simulink model "AVW_b"  (Simulink 8.7)
settings: Solver=ode1  SolverMode=SingleTasking  StartTime=0.0  StopTime=500  FixedStep=0.001  RelTol=1e-3
(part 1 of 4)
settings Model: Creator=李昊泉  LastModifiedBy=user
settings DataIOCC: LimitDataPoints=off  SaveFormat=Dataset
settings DebuggingCC: UnderspecifiedInitializationDetection=Simplified  MergeDetectMultiDrivingBlocksExec=error  MultiTaskRateTransMsg=warning  SFUnexpectedBacktrackingDiag=error  SFNoUnconditionalDefaultTransitionDiag=error
settings HardwareCC: ProdBitPerPointer=64  ProdLargestAtomicFloat=Float  ProdIntDivRoundTo=Zero  ProdEndianess=LittleEndian  ProdWordSize=64  ProdHWDeviceType=Intel->x86-64 (Windows64)
settings ModelReferenceCC: PropagateSignalLabelsOutOfModel=on
settings GRTTargetCC: TargetLangStandard=C99 (ISO)  GeneratePreprocessorConditionals=Use local settings
settings ConfigComp: CovMetricSettings=dwe  CovHtmlReporting=off  CovSaveCumulativeToWorkspaceVar=off  CovSaveSingleToWorkspaceVar=off  CovModelRefEnable=off  CovExternalEMLEnable=on

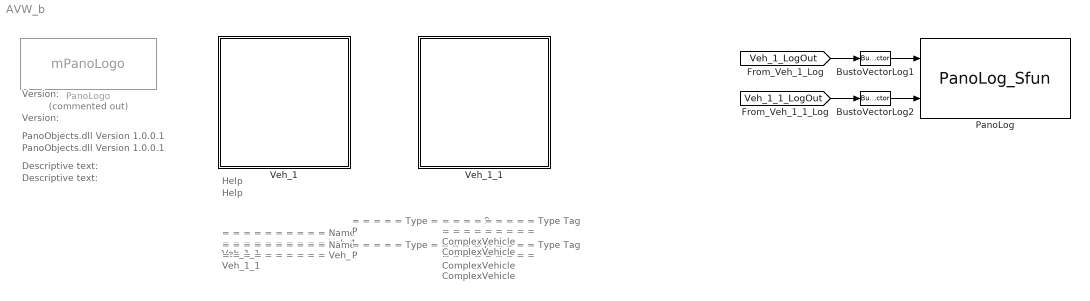
== system AVW_b ==
  note: Version:
  note: PanoObjects.dll Version 1.0.0.1
  note: Descriptive text:
  note: Help
  note: = = = = = = = = = =
      |   Name
      | = = = = = = = = = =
      |  Veh_1
      |  Veh_1_1
  note: = = = = =
      |   Type
      | = = = = =
      |   P
      |   P
  note: = = = = = = = = =
      |     Type Tag
      | = = = = = = = = =
      |  ComplexVehicle
      |  ComplexVehicle
  note: Version:
  note: PanoObjects.dll Version 1.0.0.1
  note: Descriptive text:
  note: Help
  note: = = = = = = = = = =
      |   Name
      | = = = = = = = = = =
      |  Veh_1
      |  Veh_1_1
  note: = = = = =
      |   Type
      | = = = = =
      |   P
      |   P
  note: = = = = = = = = =
      |     Type Tag
      | = = = = = = = = =
      |  ComplexVehicle
      |  ComplexVehicle
  BustoVectorLog1 : BusToVector  Tag=PanoSim_System
  BustoVectorLog2 : BusToVector  Tag=PanoSim_System
  PanoLog : S-Function  Tag=PanoSim_System  FunctionName=PanoLog_Sfun  Parameters='2','@a44ccdad-f3b7-457b-a93d-aa312d6adfaf@061ba28a-7ae2-444e-a441-87ffc9ae99f9','Matlab'  SFunctionDeploymentMode=off  EnableBusSupport=off
  PanoLogo : M-S-Function  Tag=PanoSim_System  Commented=on  FunctionName=mPanoLogo
      mask DialogControl Control2 Prompt: Welcome to use PanoSim!
      mask Display: image(imread('panosim.jpg'));
  Veh_1 : Subsystem  Tag=PanoSim_System
      mask Display: image(imread('Sedan_2.jpg'));color('white');text(0,0,'Veh_1','HorizontalAlignment','left','verticalAlignment','bottom');color('red');text(0.1,0.1,'P','HorizontalAlignment','right','verticalAlignment','top');
  Veh_1_1 : Subsystem  Tag=PanoSim_System
      mask Display: image(imread('Sedan_2.jpg'));color('white');text(0,0,'Veh_1_1','HorizontalAlignment','left','verticalAlignment','bottom');color('red');text(0.1,0.1,'P','HorizontalAlignment','right','verticalAlignment','top');
  wires:
  [Veh_1_LogOut] -> BustoVectorLog1/1
  BustoVectorLog1/1 -> PanoLog/1
  [Veh_1_1_LogOut] -> BustoVectorLog2/1
  BustoVectorLog2/1 -> PanoLog/2

== system AVW_b/Veh_1 ==
  note: = = = = = = = = = = = = = = = = = = = = = = = = = = = = = = = = =
      | English Description
      | = = = = = = = = = = = = = = = = = = = = = = = = = = = = = = = = =
      | Vehicle output bus
  note: = = = =
      | Unit
      | = = = =
  note: = = = =
      | Type
      | = = = =
      | Array
  note: = = = = = = = = = = =
      | Signal Source
      | = = = = = = = = = = =
      |  Vehicle
  note: = = = = = = = =
      | Output
      | = = = = = = = =
      |  Vehicle_out
  note: = = = = = = = = = = = = = = = = = = = = = = = = = = = = = = = = =
      | English Description
      | = = = = = = = = = = = = = = = = = = = = = = = = = = = = = = = = =
      |  throttle
      |  Gear mode, 0 neutral, 1 manual, 5 automatic ,  -1 reverse
      |  In manual mode, gear is defined by variable driver
      |  Brake master cylinder pressure
      |  Steering wheel angle
      |  wheel brake moment
      |  Wheel steering angle
  note: = = = =
      | Unit
      | = = = =
      |
      |
      |
      |  Pa
      |  rad
      |
      |  rad
  note: = = = =
      | Type
      | = = = =
      |  Single
      |  Single
      |  Single
      |  Single
      |  Single
      |  Array
      |  Array
  note: = = = = = = = = = = =
      | Signal Source
      | = = = = = = = = = = =
      |  Driver(Powertrian)
      |  Driver(Powertrian)
      |  Driver(Powertrian)
      |  Driver(Brake)
      |  Driver(Steer)
      |  Ground
      |  Ground
  note: = = = = = = = =
      | Input
      | = = = = = = = =
      |  throttle
      |  modetr
      |  geartr
      |  pcon_bk
      |  drstr_drv
      |  direc_brake
      |  direc_steer
  note: Help
  ComplexVehicleModel : Subsystem  Tag=PanoSim_System
      mask Display: image(imread('Sedan_2.jpg'));color('white');text(0,0,'Veh_1','HorizontalAlignment','left','verticalAlignment','bottom');color('red');text(0.1,0.1,'P','HorizontalAlignment','right','verticalAlignment','top');
  DriverModel : Subsystem  Tag=PanoSim_System
      mask Display: image(imread('driver.jpg'))
  Ground : Ground
  Ground1 : Ground
  Subsystem : Subsystem
  V2Sens : BusCreator  Tag=PanoSim_System  Inputs=7
  VehBusSelector1 : BusSelector  Tag=PanoSim_System  OutputSignals=Body_Out_Bus.Chassis_Motion.XO,Body_Out_Bus.Chassis_Motion.YO,Body_Out_Bus.Chassis_Motion.ZO,Body_Out_Bus.Chassis_Motion.YAW,Body_Out_Bus.Chassis_Motion.PITCH,Body_Out_Bus.Chassis_Motion.ROLL,Body_Out_Bus.Chassis_Motion.VX
  VehBusSelector2 : BusSelector  Tag=PanoSim_System  OutputSignals=Driver2Powertrain.throttle,Driver2Powertrain.modetr,Driver2Powertrain.geartr,Driver2Brake.pcon_bk,Driver2Steer.drstr_drv
  Veh_1_Sensors : Subsystem  Tag=PanoSim_System
      mask Display: image(imread('sensor.jpg'))
  tag scope: Veh_1_LogOut=global
  wires:
  Subsystem/1(PlotBuilder_out) -> [Veh_1_LogOut]
  ComplexVehicleModel/1(VehicleOut) -> Subsystem/1(VehicleDynOut), [VehicleDynOut], VehBusSelector1/1  "Vehicle_Out"
  V2Sens/1 -> [VehicleOut], Veh_1_Sensors/1(In1)
  VehBusSelector2/1 -> ComplexVehicleModel/1(Throttle)  "<throttle>"
  VehBusSelector2/5 -> ComplexVehicleModel/5(SteerAngle)  "<drstr_drv>"
  DriverModel/1(DriverOut) -> VehBusSelector2/1
  VehBusSelector1/1 -> V2Sens/1  "<XO>"
  [VehicleDynOut] -> DriverModel/1(VehicleInput)
  Ground/1 -> ComplexVehicleModel/6(Direct Brake)
  VehBusSelector1/3 -> V2Sens/3  "<ZO>"
  VehBusSelector1/4 -> V2Sens/4  "<YAW>"
  VehBusSelector1/2 -> V2Sens/2  "<YO>"
  VehBusSelector1/7 -> V2Sens/7  "<VX>"
  Ground1/1 -> ComplexVehicleModel/7(Direct Steer)
  VehBusSelector1/6 -> V2Sens/6  "<ROLL>"
  VehBusSelector2/4 -> ComplexVehicleModel/4(BrakeControl)  "<pcon_bk>"
  VehBusSelector1/5 -> V2Sens/5  "<PITCH>"
  VehBusSelector2/3 -> ComplexVehicleModel/3(Gear)  "<geartr>"
  VehBusSelector2/2 -> ComplexVehicleModel/2(TransMode)  "<modetr>"

== system AVW_b/Veh_1_1 ==
  note: = = = = = = = = = = = = = = = = = = = = = = = = = = = = = = = = =
      | English Description
      | = = = = = = = = = = = = = = = = = = = = = = = = = = = = = = = = =
      | Vehicle output bus
  note: = = = =
      | Unit
      | = = = =
  note: = = = =
      | Type
      | = = = =
      | Array
  note: = = = = = = = = = = =
      | Signal Source
      | = = = = = = = = = = =
      |  Vehicle
  note: = = = = = = = =
      | Output
      | = = = = = = = =
      |  Vehicle_out
  note: = = = = = = = = = = = = = = = = = = = = = = = = = = = = = = = = =
      | English Description
      | = = = = = = = = = = = = = = = = = = = = = = = = = = = = = = = = =
      |  throttle
      |  Gear mode, 0 neutral, 1 manual, 5 automatic ,  -1 reverse
      |  In manual mode, gear is defined by variable driver
      |  Brake master cylinder pressure
      |  Steering wheel angle
      |  wheel brake moment
      |  Wheel steering angle
  note: = = = =
      | Unit
      | = = = =
      |
      |
      |
      |  Pa
      |  rad
      |
      |  rad
  note: = = = =
      | Type
      | = = = =
      |  Single
      |  Single
      |  Single
      |  Single
      |  Single
      |  Array
      |  Array
  note: = = = = = = = = = = =
      | Signal Source
      | = = = = = = = = = = =
      |  Driver(Powertrian)
      |  Driver(Powertrian)
      |  Driver(Powertrian)
      |  Driver(Brake)
      |  Driver(Steer)
      |  Ground
      |  Ground
  note: = = = = = = = =
      | Input
      | = = = = = = = =
      |  throttle
      |  modetr
      |  geartr
      |  pcon_bk
      |  drstr_drv
      |  direc_brake
      |  direc_steer
  note: Help
  ComplexVehicleModel : Subsystem  Tag=PanoSim_System
      mask Display: image(imread('Sedan_2.jpg'));color('white');text(0,0,'Veh_1_1','HorizontalAlignment','left','verticalAlignment','bottom');color('red');text(0.1,0.1,'P','HorizontalAlignment','right','verticalAlignment','top');
  DriverModel : Subsystem  Tag=PanoSim_System
      mask Display: image(imread('driver.jpg'))
  Ground : Ground
  Ground1 : Ground
  Subsystem : Subsystem
  V2Sens : BusCreator  Tag=PanoSim_System  Inputs=7
  VehBusSelector1 : BusSelector  Tag=PanoSim_System  OutputSignals=Body_Out_Bus.Chassis_Motion.XO,Body_Out_Bus.Chassis_Motion.YO,Body_Out_Bus.Chassis_Motion.ZO,Body_Out_Bus.Chassis_Motion.YAW,Body_Out_Bus.Chassis_Motion.PITCH,Body_Out_Bus.Chassis_Motion.ROLL,Body_Out_Bus.Chassis_Motion.VX
  VehBusSelector2 : BusSelector  Tag=PanoSim_System  OutputSignals=Driver2Powertrain.throttle,Driver2Powertrain.modetr,Driver2Powertrain.geartr,Driver2Brake.pcon_bk,Driver2Steer.drstr_drv
  Veh_1_1_Sensors : Subsystem  Tag=PanoSim_System
      mask Display: image(imread('sensor.jpg'))
  tag scope: Veh_1_1_LogOut=global
  wires:
  Subsystem/1(PlotBuilder_out) -> [Veh_1_1_LogOut]
  ComplexVehicleModel/1(VehicleOut) -> Subsystem/1(VehicleDynOut), [VehicleDynOut], VehBusSelector1/1  "Vehicle_Out"
  V2Sens/1 -> [VehicleOut], Veh_1_1_Sensors/1(In1)
  VehBusSelector2/1 -> ComplexVehicleModel/1(Throttle)  "<throttle>"
  VehBusSelector2/5 -> ComplexVehicleModel/5(SteerAngle)  "<drstr_drv>"
  DriverModel/1(DriverOut) -> VehBusSelector2/1
  VehBusSelector1/1 -> V2Sens/1  "<XO>"
  [VehicleDynOut] -> DriverModel/1(VehicleInput)
  Ground/1 -> ComplexVehicleModel/6(Direct Brake)
  VehBusSelector1/3 -> V2Sens/3  "<ZO>"
  VehBusSelector1/4 -> V2Sens/4  "<YAW>"
  VehBusSelector1/2 -> V2Sens/2  "<YO>"
  VehBusSelector1/7 -> V2Sens/7  "<VX>"
  Ground1/1 -> ComplexVehicleModel/7(Direct Steer)
  VehBusSelector1/6 -> V2Sens/6  "<ROLL>"
  VehBusSelector2/4 -> ComplexVehicleModel/4(BrakeControl)  "<pcon_bk>"
  VehBusSelector1/5 -> V2Sens/5  "<PITCH>"
  VehBusSelector2/3 -> ComplexVehicleModel/3(Gear)  "<geartr>"
  VehBusSelector2/2 -> ComplexVehicleModel/2(TransMode)  "<modetr>"

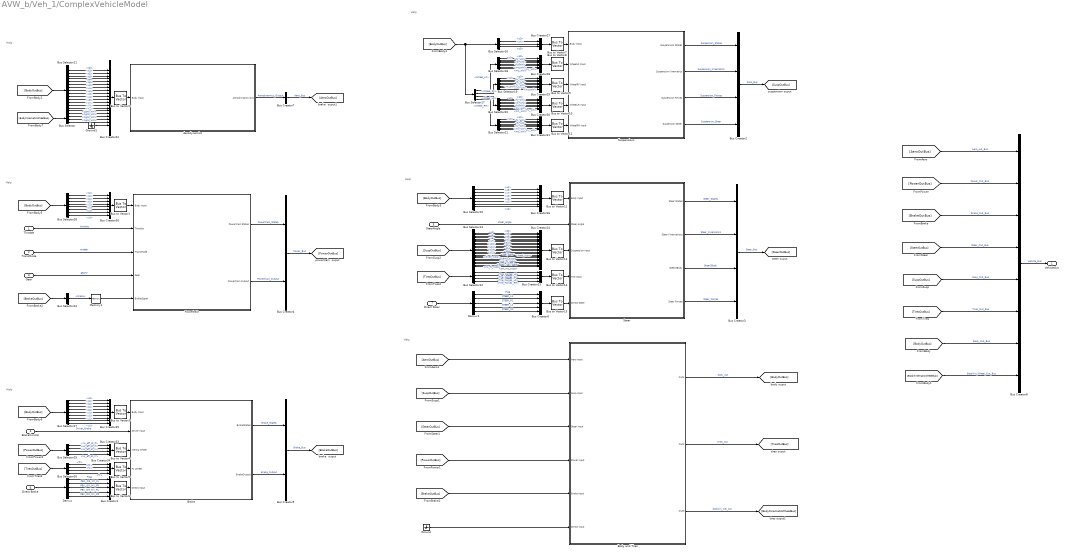
== system AVW_b/Veh_1/ComplexVehicleModel ==
  note: Help
  note: Help
  note: Help
  note: Help
  note: Help
  note: Help
  Throttle : Inport
  TransMode : Inport  Port=2
  Gear : Inport  Port=3
  BrakeControl : Inport  Port=4
  SteerAngle : Inport  Port=5
  Direct Brake : Inport  Port=6
  Direct Steer : Inport  Port=7
  Aerodynamics : Subsystem
  Body and Tires : Subsystem
  Brake : Subsystem
  Bus Creator1 : BusCreator  Inputs=5
  Bus Creator{2..3,23,33..34} (5 alike) : BusCreator  Inputs=4
  Bus Creator22 : BusCreator  Inputs=20
  Bus Creator24 : BusCreator  Inputs=24
  Bus Creator26 : BusCreator  Inputs=7
  Bus Creator27 : BusCreator  Inputs=3
  Bus Creator{8,28..31,36} (6 alike) : BusCreator  Inputs=8
  Bus Creator35 : BusCreator  Inputs=9
  Bus Creator4 : BusCreator  Inputs=2
  Bus Creator5 : BusCreator  Inputs=2
  Bus Creator6 : BusCreator  Inputs=5
  Bus Creator7 : BusCreator  Inputs=1
  Bus Selector : BusSelector  OutputSignals=bodykin_whl_out_lf.zgnd_whl,bodykin_whl_out_rf.zgnd_whl,bodykin_whl_out_lr.zgnd_whl,bodykin_whl_out_rr.zgnd_whl
  Bus Selector11 : BusSelector  OutputSignals=Chassi_States.q0,Chassi_States.q1,Chassi_States.q2,Chassi_States.q3,Chassi_States.q4,Chassi_States.q5,Chassi_States.u0,Chassi_States.u1,Chassi_States.u2,Chassi_States.u3,Chassi_States.u4,Chassi_States.u5,Chassis_Motion.VX,Chassis_Motion.VY,Chassis_Motion.VZ
  Bus Selector12 : BusSelector  OutputSignals=Tire_Forces_LF,Tire_Forces_RF,Tire_Forces_LR,Tire_Forces_RR
  Bus Selector13 : BusSelector  OutputSignals=Suspension_States.q2,Suspension_States.u2,Suspension_States.q3,Suspension_States.u3,Suspension_States.q6,Suspension_States.u6,Suspension_States.q7,Suspension_States.u7,Suspension_States.q10,Suspension_States.u10,Suspension_States.q11,Suspension_States.u11,Suspension_States.q14,Suspension_States.u14,Suspension_States.q15,Suspension_States.u15,Suspension_Kinematics.toe_susp,Suspension_Kinematics.toed_susp,Suspension_Kinematics.dived_susp,Suspension_Kinematics.camd_susp,Suspension_Kinematics.dcam_con_susp,Suspension_Steer.sw_fx_susp,Suspension_Steer.sw_fy_susp,Suspension_Steer.sw_mz_susp
  Bus Selector15 : BusSelector  OutputSignals=Chassi_States.u0,Chassi_States.u6,Chassi_States.u7,Wheel_LF.u0,Wheel_RF.u0,Wheel_LR.u0,Wheel_RR.u0
  Bus Selector16 : BusSelector  OutputSignals=Chassi_States.u3,Chassi_States.u4,Chassi_States.u5
  Bus Selector17 : BusSelector  OutputSignals=Wheel_LF,Wheel_RF,Wheel_LR,Wheel_RR
  Bus Selector{18..21} (4 alike) : BusSelector  OutputSignals=q0,u0,fx_whl,fy_whl,fz_whl,mx_whl,my_whl,mz_whl
  Bus Selector23 : BusSelector  OutputSignals=Brake_Output.brake
  Bus Selector25 : BusSelector  OutputSignals=Powertrain_Output.iw_eff_pt_lf,Powertrain_Output.iw_eff_pt_rf,Powertrain_Output.iw_eff_pt_lr,Powertrain_Output.iw_eff_pt_rr
  Bus Selector26 : BusSelector  OutputSignals=Tire_Forces_LF.fz,Tire_Forces_RF.fz,Tire_Forces_LR.fz,Tire_Forces_RR.fz
  Bus Selector27 : BusSelector  OutputSignals=Chassi_States.u0,Wheel_LF.q1,Wheel_RF.q1,Wheel_LR.q1,Wheel_RR.q1,Wheel_LF.u1,Wheel_RF.u1,Wheel_LR.u1,Wheel_RR.u1
  Bus Selector28 : BusSelector  OutputSignals=Wheel_LF.q1,Wheel_RF.q1,Wheel_LR.q1,Wheel_RR.q1,Wheel_LF.u1,Wheel_RF.u1,Wheel_LR.u1,Wheel_RR.u1
  Bus to Vector{1..15} (15 alike) : BusToVector
  Demux : Demux  Outputs=5
  Demux1 : Demux  Outputs=5
  Ground : Ground
  Ground1 : Ground
  Memory1 : Memory
  Powertrain : Subsystem
  Steer : Subsystem
  Suspensions : Subsystem
  VehicleOut : Outport
  wires:
  Ground/1 -> Body and Tires/6(Direct Input)
  Bus Selector13/24 -> Bus Creator24/24  "<sw_mz_susp>"
  Bus Selector13/23 -> Bus Creator24/23  "<sw_fy_susp>"
  Bus Selector13/22 -> Bus Creator24/22  "<sw_fx_susp>"
  Bus Selector13/21 -> Bus Creator24/21  "<dcam_con_susp>"
  Bus Selector13/20 -> Bus Creator24/20  "<camd_susp>"
  Bus Selector13/19 -> Bus Creator24/19  "<dived_susp>"
  Bus Selector13/18 -> Bus Creator24/18  "<toed_susp>"
  Bus Selector13/17 -> Bus Creator24/17  "<toe_susp>"
  Bus Selector13/16 -> Bus Creator24/16  "<u15>"
  Bus Selector13/15 -> Bus Creator24/15  "<q15>"
  Bus Selector13/14 -> Bus Creator24/14  "<u14>"
  Bus Selector13/13 -> Bus Creator24/13  "<q14>"
  Bus Selector13/12 -> Bus Creator24/12  "<u11>"
  Bus Selector13/11 -> Bus Creator24/11  "<q11>"
  Bus Selector13/10 -> Bus Creator24/10  "<u10>"
  Bus Selector13/9 -> Bus Creator24/9  "<q10>"
  Bus Selector13/8 -> Bus Creator24/8  "<u7>"
  Bus Selector13/7 -> Bus Creator24/7  "<q7>"
  Bus Selector13/6 -> Bus Creator24/6  "<u6>"
  Bus Selector13/5 -> Bus Creator24/5  "<q6>"
  Bus Selector13/4 -> Bus Creator24/4  "<u3>"
  Bus Selector13/3 -> Bus Creator24/3  "<q3>"
  Bus Selector13/2 -> Bus Creator24/2  "<u2>"
  Bus Selector13/1 -> Bus Creator24/1  "<q2>"
  Demux1/5 -> Bus Creator6/5  "STEER_R2"
  Demux1/4 -> Bus Creator6/4  "STEER_L2"
  Demux1/3 -> Bus Creator6/3  "STEER_R1"
  Demux1/2 -> Bus Creator6/2  "STEER_L1"
  Demux1/1 -> Bus Creator6/1  "Flag"
  Direct Steer/1 -> Demux1/1
  Bus Creator6/1 -> Bus to Vector15/1
  Demux/5 -> Bus Creator1/5  "PBK_OR_MY_RR"
  Demux/4 -> Bus Creator1/4  "PBK_OR_MY_RL"
  Demux/3 -> Bus Creator1/3  "PBK_OR_MY_FR"
  Demux/2 -> Bus Creator1/2  "PBK_OR_MY_FL"
  Demux/1 -> Bus Creator1/1  "Flag"
  Direct Brake/1 -> Demux/1
  SteerAngle/1 -> Steer/2(Steer Angle)  "steer_angle"
  [TiresOutBus] -> Bus Creator8/6  "Tires_Out_Bus"
  [SuspOutBus] -> Bus Creator8/5  "Susp_Out_Bus"
  [SteerOutBus] -> Bus Creator8/4  "Steer_Out_Bus"
  [BrakeOutBus] -> Bus Creator8/3  "Brake_Out_Bus"
  [PowerOutBus] -> Bus Creator8/2  "Power_Out_BUs"
  [AeroOutBus] -> Bus Creator8/1  "Aero_out_Bus"
  Suspensions/4(Suspension Steer) -> Bus Creator2/4  "Suspension_Steer"
  Suspensions/3(Suspension Forces) -> Bus Creator2/3  "Suspension_Forces"
  Suspensions/1(Suspensions States) -> Bus Creator2/1  "Suspension_States"
  Suspensions/2(Suspension Kinematics) -> Bus Creator2/2  "Suspension_Kinematics"
  Bus Creator2/1 -> [SuspOutBus]  "Susp_Bus"
  Steer/1(Steer States) -> Bus Creator3/1  "Steer_States"
  Steer/2(Steer Kinematiocs) -> Bus Creator3/2  "Steer_Kinematics"
  Steer/3(Steer2Body) -> Bus Creator3/3  "Steer2Body"
  Steer/4(Steer Forces) -> Bus Creator3/4  "Steer_Forces"
  Bus Creator3/1 -> [SteerOutBus]  "Steer_Bus"
  Powertrain/1(Powertrain States) -> Bus Creator4/1  "Powertrain_States"
  Powertrain/2(Powertrain Output) -> Bus Creator4/2  "Powertrain_Output"
  Bus Creator4/1 -> [PowerOutBus]  "Power_Bus"
  Brake/1(BrakeStates) -> Bus Creator5/1  "Brake_States"
  Brake/2(BrakeOutput) -> Bus Creator5/2  "Brake_Output"
  Bus Creator5/1 -> [BrakeOutBus]  "Brake_Bus"
  Aerodynamics/1(Aerodymatics Out) -> Bus Creator7/1  "Aerodynamics_Output"
  Bus Creator7/1 -> [AeroOutBus]  "Aero_Bus"
  Bus Creator8/1 -> VehicleOut/1  "Vehicle_Bus"
  [BodyOutBus] -> Bus Creator8/7  "Body_Out_Bus"
  [BodyOutBus] -> Bus Selector11/1
  [TiresOutBus] -> Bus Selector12/1
  Bus Selector12/1 -> Bus Creator23/1  "<Tire_Forces_LF>"
  Bus Selector12/2 -> Bus Creator23/2  "<Tire_Forces_RF>"
  Bus Selector12/3 -> Bus Creator23/3  "<Tire_Forces_LR>"
  Bus Selector12/4 -> Bus Creator23/4  "<Tire_Forces_RR>"
  [SuspOutBus] -> Bus Selector13/1
  Bus Creator24/1 -> Bus to Vector13/1
  [BodyOutBus] -> Bus Selector15/1
  Bus Selector15/1 -> Bus Creator26/1  "<u0>"
  Bus Selector15/2 -> Bus Creator26/2  "<u6>"
  Bus Selector15/3 -> Bus Creator26/3  "<u7>"
  Bus Selector15/4 -> Bus Creator26/4  "<u0>"
  Bus Selector15/5 -> Bus Creator26/5  "<u0>"
  Bus Selector15/6 -> Bus Creator26/6  "<u0>"
  Bus Selector15/7 -> Bus Creator26/7  "<u0>"
  Bus Selector16/1 -> Bus Creator27/1  "<u3>"
  Bus Selector16/2 -> Bus Creator27/2  "<u4>"
  Bus Selector16/3 -> Bus Creator27/3  "<u5>"
  Bus Creator27/1 -> Bus to Vector7/1
  Bus Selector17/1 -> Bus Selector18/1  "<Wheel_LF>"
  Bus Selector18/1 -> Bus Creator28/1  "<q0>"
  Bus Selector18/2 -> Bus Creator28/2  "<u0>"
  Bus Selector18/3 -> Bus Creator28/3  "<fx_whl>"
  Bus Selector18/4 -> Bus Creator28/4  "<fy_whl>"
  Bus Selector18/5 -> Bus Creator28/5  "<fz_whl>"
  Bus Selector18/6 -> Bus Creator28/6  "<mx_whl>"
  Bus Selector18/7 -> Bus Creator28/7  "<my_whl>"
  Bus Selector18/8 -> Bus Creator28/8  "<mz_whl>"
  Bus Selector19/1 -> Bus Creator29/1  "<q0>"
  Bus Selector19/2 -> Bus Creator29/2  "<u0>"
  Bus Selector19/3 -> Bus Creator29/3  "<fx_whl>"
  Bus Selector19/4 -> Bus Creator29/4  "<fy_whl>"
  Bus Selector19/5 -> Bus Creator29/5  "<fz_whl>"
  Bus Selector19/6 -> Bus Creator29/6  "<mx_whl>"
  Bus Selector19/7 -> Bus Creator29/7  "<my_whl>"
  Bus Selector19/8 -> Bus Creator29/8  "<mz_whl>"
  Bus Selector20/1 -> Bus Creator30/1  "<q0>"
  Bus Selector20/2 -> Bus Creator30/2  "<u0>"
  Bus Selector20/3 -> Bus Creator30/3  "<fx_whl>"
  Bus Selector20/4 -> Bus Creator30/4  "<fy_whl>"
  Bus Selector20/5 -> Bus Creator30/5  "<fz_whl>"
  Bus Selector20/6 -> Bus Creator30/6  "<mx_whl>"
  Bus Selector20/7 -> Bus Creator30/7  "<my_whl>"
  Bus Selector20/8 -> Bus Creator30/8  "<mz_whl>"
  Bus Selector21/1 -> Bus Creator31/1  "<q0>"
  Bus Selector21/2 -> Bus Creator31/2  "<u0>"
  Bus Selector21/3 -> Bus Creator31/3  "<fx_whl>"
  Bus Selector21/4 -> Bus Creator31/4  "<fy_whl>"
  Bus Selector21/5 -> Bus Creator31/5  "<fz_whl>"
  Bus Selector21/6 -> Bus Creator31/6  "<mx_whl>"
  Bus Selector21/7 -> Bus Creator31/7  "<my_whl>"
  Bus Selector21/8 -> Bus Creator31/8  "<mz_whl>"
  Bus Selector17/2 -> Bus Selector19/1  "<Wheel_RF>"
  Bus Selector17/3 -> Bus Selector20/1  "<Wheel_LR>"
  Bus Selector17/4 -> Bus Selector21/1  "<Wheel_RR>"
  Bus Creator28/1 -> Bus to Vector8/1
  Bus Creator29/1 -> Bus to Vector9/1
  Bus Creator30/1 -> Bus to Vector10/1
  Bus Creator31/1 -> Bus to Vector11/1
  Throttle/1 -> Powertrain/2(Throttle)  "throttle"
  TransMode/1 -> Powertrain/3(TransMode)  "modetr"
  Gear/1 -> Powertrain/4(Gear)  "geartr"
  [BrakeOutBus] -> Bus Selector23/1
  BrakeControl/1 -> Brake/2(Driver Input)  "Driver_Brake"
  [PowerOutBus] -> Bus Selector25/1
  Bus Selector25/1 -> Bus Creator33/1  "<iw_eff_pt_lf>"
  Bus Selector25/2 -> Bus Creator33/2  "<iw_eff_pt_rf>"
  Bus Selector25/3 -> Bus Creator33/3  "<iw_eff_pt_lr>"
  Bus Selector25/4 -> Bus Creator33/4  "<iw_eff_pt_rr>"
  [TiresOutBus] -> Bus Selector26/1
  Bus Selector26/1 -> Bus Creator34/1  "<fz>"
  Bus Selector26/2 -> Bus Creator34/2  "<fz>"
  Bus Selector26/3 -> Bus Creator34/3  "<fz>"
  Bus Selector26/4 -> Bus Creator34/4  "<fz>"
  [BodyOutBus] -> Bus Selector27/1
  Bus Selector27/1 -> Bus Creator35/1  "<u0>"
  Bus Selector27/2 -> Bus Creator35/2  "<q1>"
  Bus Selector27/3 -> Bus Creator35/3  "<q1>"
  Bus Selector27/4 -> Bus Creator35/4  "<q1>"
  Bus Selector27/5 -> Bus Creator35/5  "<q1>"
  Bus Selector27/6 -> Bus Creator35/6  "<u1>"
  Bus Selector27/7 -> Bus Creator35/7  "<u1>"
  Bus Selector27/8 -> Bus Creator35/8  "<u1>"
  Bus Selector27/9 -> Bus Creator35/9  "<u1>"
  [BodyOutBus] -> Bus Selector28/1
  Bus Selector28/1 -> Bus Creator36/1  "<q1>"
  Bus Selector28/2 -> Bus Creator36/2  "<q1>"
  Bus Selector28/3 -> Bus Creator36/3  "<q1>"
  Bus Selector28/4 -> Bus Creator36/4  "<q1>"
  Bus Selector28/5 -> Bus Creator36/5  "<u1>"
  Bus Selector28/6 -> Bus Creator36/6  "<u1>"
  Bus Selector28/7 -> Bus Creator36/7  "<u1>"
  Bus Selector28/8 -> Bus Creator36/8  "<u1>"
  Bus Selector11/1 -> Bus Creator22/1  "<q0>"
  Bus Selector11/2 -> Bus Creator22/2  "<q1>"
  Bus Selector11/3 -> Bus Creator22/3  "<q2>"
  Bus Selector11/4 -> Bus Creator22/4  "<q3>"
  Bus Selector11/5 -> Bus Creator22/5  "<q4>"
  Bus Selector11/6 -> Bus Creator22/6  "<q5>"
  Bus Selector11/7 -> Bus Creator22/7  "<u0>"
  Bus Selector11/8 -> Bus Creator22/8  "<u1>"
  Bus Selector11/9 -> Bus Creator22/9  "<u2>"
  Bus Selector11/10 -> Bus Creator22/10  "<u3>"
  Bus Selector11/11 -> Bus Creator22/11  "<u4>"
  Bus Selector11/12 -> Bus Creator22/12  "<u5>"
  Bus Selector11/13 -> Bus Creator22/13  "<VX>"
  Bus Selector11/14 -> Bus Creator22/14  "<VY>"
  Bus Selector11/15 -> Bus Creator22/15  "<VZ>"
  Ground1/1 -> Bus Creator22/20
  [SteerOutBus] -> Body and Tires/3(Steer Input)
  [PowerOutBus] -> Body and Tires/4(Power Input)
  Body and Tires/1(Out1) -> [BodyOutBus]  "body_out"
  Body and Tires/2(Out2) -> [TiresOutBus]  "tires_out"
  [AeroOutBus] -> Body and Tires/1(Aero Input)
  [SuspOutBus] -> Body and Tires/2(Susp Input)
  Bus Selector23/1 -> Memory1/1  "<brake>"
  Memory1/1 -> Powertrain/5(BrakeSignal)
  Bus Creator26/1 -> Bus to Vector12/1
  Bus Creator23/1 -> Bus to Vector14/1
  Bus Creator36/1 -> Bus to Vector1/1
  [BodyOutBus] -> Bus Selector16/1, Bus Selector17/1
  [BrakeOutBus] -> Body and Tires/5(Brake Input)
  Body and Tires/3(Out3) -> [BodyKinematicWheelBus]  "bodykin_wel_out"
  [BodyKinematicWheelBus] -> Bus Creator8/8  "BodyKin_Wheel_Out_Bus"
  [BodyKinematicWheelBus] -> Bus Selector/1
  Bus Selector/1 -> Bus Creator22/16  "<zgnd_whl>"
  Bus Selector/2 -> Bus Creator22/17  "<zgnd_whl>"
  Bus Selector/3 -> Bus Creator22/18  "<zgnd_whl>"
  Bus Selector/4 -> Bus Creator22/19  "<zgnd_whl>"
  Bus Creator22/1 -> Bus to Vector2/1
  Bus to Vector2/1 -> Aerodynamics/1(Body Input)
  Bus to Vector1/1 -> Powertrain/1(Body Input)
  Bus Creator35/1 -> Bus to Vector3/1
  Bus to Vector3/1 -> Brake/1(Body Input)
  Bus Creator33/1 -> Bus to Vector4/1
  Bus to Vector4/1 -> Brake/3(Inertia Wheel)
  Bus Creator34/1 -> Bus to Vector5/1
  Bus to Vector5/1 -> Brake/4(Fz Wheel)
  Bus Creator1/1 -> Bus to Vector6/1
  Bus to Vector6/1 -> Brake/5(Direct Input)
  Bus to Vector7/1 -> Suspensions/1(Body Input)
  Bus to Vector8/1 -> Suspensions/2(WheelLF Input)
  Bus to Vector9/1 -> Suspensions/3(WheelRF Input)
  Bus to Vector10/1 -> Suspensions/4(WheelLR Input)
  Bus to Vector11/1 -> Suspensions/5(WheelRR Input)
  Bus to Vector12/1 -> Steer/1(Body Input)
  Bus to Vector13/1 -> Steer/3(Suspension Input)
  Bus to Vector14/1 -> Steer/4(Tire Input)
  Bus to Vector15/1 -> Steer/5(Direct Steer)

== system AVW_b/Veh_1/DriverModel ==
  note: Help
  VehicleInput : Inport
  Bus Creator37 : BusCreator  Inputs=10
  Bus Creator38 : BusCreator  Inputs=2
  Bus Creator39 : BusCreator  Inputs=2
  Bus Creator6 : BusCreator  Inputs=4
  Bus Selector : BusSelector  OutputSignals=Body_Out_Bus,Steer_Out_Bus,Power_Out_BUs,Brake_Out_Bus
  Bus Selector29 : BusSelector  OutputSignals=Chassi_States.q0,Chassi_States.q1,Chassi_States.q3,Chassi_States.u0,Chassi_States.u1,Chassi_States.u3,Wheel_LF.u1,Wheel_RF.u1,Wheel_LR.u1,Wheel_RR.u1
  Bus Selector30 : BusSelector  OutputSignals=Steer_Kinematics.str_sus_f,Steer_Kinematics.str_sus_r
  Bus Selector31 : BusSelector  OutputSignals=Powertrain_Output.av_eng,Powertrain_Output.aa_eng
  Bus Selector32 : BusSelector  OutputSignals=Brake_Output.turn_off
  Driver : Subsystem
  DriverOut : Outport
  wires:
  Bus Creator6/1 -> DriverOut/1  "Driver_Bus"
  Bus Creator39/1 -> Driver/3(Engine Input)
  Bus Selector31/2 -> Bus Creator39/2  "<aa_eng>"
  Bus Selector31/1 -> Bus Creator39/1  "<av_eng>"
  Bus Selector/3 -> Bus Selector31/1  "<Power_Out_BUs>"
  Bus Selector32/1 -> Driver/4(Brake Input)  "<turn_off>"
  Bus Creator38/1 -> Driver/2(Steer Input)
  Bus Selector30/2 -> Bus Creator38/2  "<str_sus_r>"
  Bus Selector30/1 -> Bus Creator38/1  "<str_sus_f>"
  Bus Selector/2 -> Bus Selector30/1  "<Steer_Out_Bus>"
  Bus Selector29/10 -> Bus Creator37/10  "<u1>"
  Bus Selector29/9 -> Bus Creator37/9  "<u1>"
  Bus Selector29/8 -> Bus Creator37/8  "<u1>"
  Bus Selector29/7 -> Bus Creator37/7  "<u1>"
  Bus Selector29/6 -> Bus Creator37/6  "<u3>"
  Bus Selector29/5 -> Bus Creator37/5  "<u1>"
  Bus Selector29/4 -> Bus Creator37/4  "<u0>"
  Bus Selector29/3 -> Bus Creator37/3  "<q3>"
  Bus Selector29/2 -> Bus Creator37/2  "<q1>"
  Bus Selector29/1 -> Bus Creator37/1  "<q0>"
  Bus Creator37/1 -> Driver/1(Body Input)
  Bus Selector/1 -> Bus Selector29/1  "<Body_Out_Bus>"
  Driver/4(Driver_Brake) -> Bus Creator6/4
  Driver/3(Driver_Powertrain) -> Bus Creator6/3
  Driver/2(Driver_Steer) -> Bus Creator6/2
  Driver/1(Driver_States) -> Bus Creator6/1
  VehicleInput/1 -> Bus Selector/1
  Bus Selector/4 -> Bus Selector32/1  "<Brake_Out_Bus>"

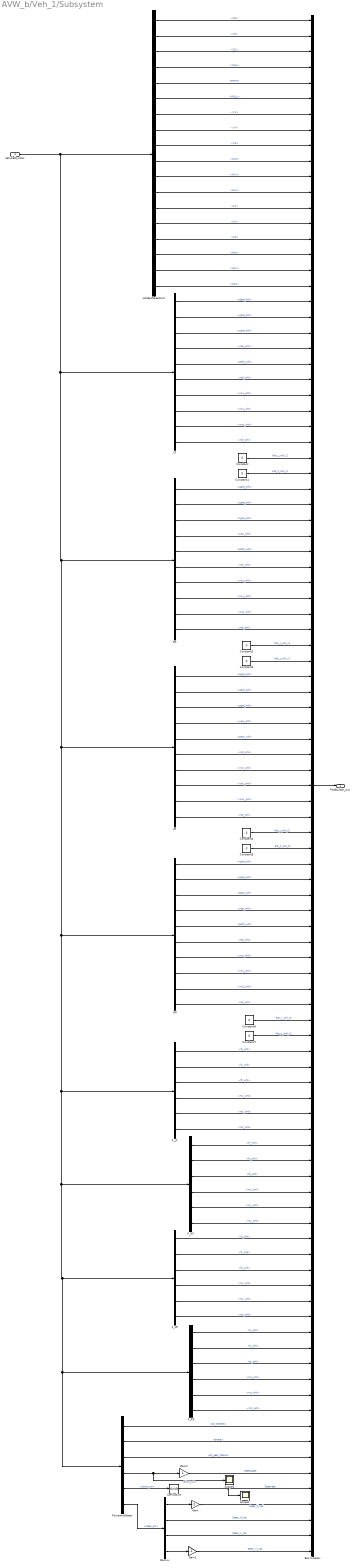
== system AVW_b/Veh_1/Subsystem ==
  VehicleDynOut : Inport
  Bus Creator : BusCreator  Inputs=99
  Constant{,1..7} (8 alike) : Constant  Value=0
  Demux : Demux
  Derivative : Derivative
  F_LF : BusSelector  Tag=PanoSim_System  OutputSignals=Body_Out_Bus.Wheel_LF.fx_whl,Body_Out_Bus.Wheel_LF.fy_whl,Body_Out_Bus.Wheel_LF.fz_whl,Body_Out_Bus.Wheel_LF.mx_whl,Body_Out_Bus.Wheel_LF.my_whl,Body_Out_Bus.Wheel_LF.mz_whl
  F_LR : BusSelector  Tag=PanoSim_System  OutputSignals=Body_Out_Bus.Wheel_LR.fx_whl,Body_Out_Bus.Wheel_LR.fy_whl,Body_Out_Bus.Wheel_LR.fz_whl,Body_Out_Bus.Wheel_LR.mx_whl,Body_Out_Bus.Wheel_LR.my_whl,Body_Out_Bus.Wheel_LR.mz_whl
  F_RF : BusSelector  Tag=PanoSim_System  OutputSignals=Body_Out_Bus.Wheel_RF.fx_whl,Body_Out_Bus.Wheel_RF.fy_whl,Body_Out_Bus.Wheel_RF.fz_whl,Body_Out_Bus.Wheel_RF.mx_whl,Body_Out_Bus.Wheel_RF.my_whl,Body_Out_Bus.Wheel_RF.mz_whl
  F_RR : BusSelector  Tag=PanoSim_System  OutputSignals=Body_Out_Bus.Wheel_RR.fx_whl,Body_Out_Bus.Wheel_RR.fy_whl,Body_Out_Bus.Wheel_RR.fz_whl,Body_Out_Bus.Wheel_RR.mx_whl,Body_Out_Bus.Wheel_RR.my_whl,Body_Out_Bus.Wheel_RR.mz_whl
  Gain : Gain  Gain=-1
  Gain1 : Gain  Gain=-1
  Gain2 : Gain
  LF : BusSelector  Tag=PanoSim_System  OutputSignals=BodyKin_Wheel_Out_Bus.bodykin_whl_out_lf.xgnd_whl,BodyKin_Wheel_Out_Bus.bodykin_whl_out_lf.ygnd_whl,BodyKin_Wheel_Out_Bus.bodykin_whl_out_lf.zgnd_whl,BodyKin_Wheel_Out_Bus.bodykin_whl_out_lf.yaw_whl,BodyKin_Wheel_Out_Bus.bodykin_whl_out_lf.pitch_whl,BodyKin_Wheel_Out_Bus.bodykin_whl_out_lf.roll_whl,BodyKin_Wheel_Out_Bus.bodykin_whl_out_lf.vwx_whl,BodyKin_Wheel_Out_Bus.bodykin_whl_out_lf.vwy_whl,BodyKin_Wheel_Out_Bus.bodykin_whl_out_lf.vwz_whl,BodyKin_Wheel_Out_Bus.bodykin_whl_out_lf.rot_whl
  LR : BusSelector  Tag=PanoSim_System  OutputSignals=BodyKin_Wheel_Out_Bus.bodykin_whl_out_lr.xgnd_whl,BodyKin_Wheel_Out_Bus.bodykin_whl_out_lr.ygnd_whl,BodyKin_Wheel_Out_Bus.bodykin_whl_out_lr.zgnd_whl,BodyKin_Wheel_Out_Bus.bodykin_whl_out_lr.yaw_whl,BodyKin_Wheel_Out_Bus.bodykin_whl_out_lr.pitch_whl,BodyKin_Wheel_Out_Bus.bodykin_whl_out_lr.roll_whl,BodyKin_Wheel_Out_Bus.bodykin_whl_out_lr.vwx_whl,BodyKin_Wheel_Out_Bus.bodykin_whl_out_lr.vwy_whl,BodyKin_Wheel_Out_Bus.bodykin_whl_out_lr.vwz_whl,BodyKin_Wheel_Out_Bus.bodykin_whl_out_lr.rot_whl
  PowerandSteer : BusSelector  Tag=PanoSim_System  OutputSignals=Power_Out_BUs.Powertrain_Output.pt_throttle,Brake_Out_Bus.Brake_Output.brake,Power_Out_BUs.Powertrain_Output.pt_gear_status,Steer_Out_Bus.Steer_Kinematics.strav_sw,Steer_Out_Bus.Steer_Kinematics.strav_sw,Steer_Out_Bus.Steer_Kinematics.steer_str
  RF : BusSelector  Tag=PanoSim_System  OutputSignals=BodyKin_Wheel_Out_Bus.bodykin_whl_out_rf.xgnd_whl,BodyKin_Wheel_Out_Bus.bodykin_whl_out_rf.ygnd_whl,BodyKin_Wheel_Out_Bus.bodykin_whl_out_rf.zgnd_whl,BodyKin_Wheel_Out_Bus.bodykin_whl_out_rf.yaw_whl,BodyKin_Wheel_Out_Bus.bodykin_whl_out_rf.pitch_whl,BodyKin_Wheel_Out_Bus.bodykin_whl_out_rf.roll_whl,BodyKin_Wheel_Out_Bus.bodykin_whl_out_rf.vwx_whl,BodyKin_Wheel_Out_Bus.bodykin_whl_out_rf.vwy_whl,BodyKin_Wheel_Out_Bus.bodykin_whl_out_rf.vwz_whl,BodyKin_Wheel_Out_Bus.bodykin_whl_out_rf.rot_whl
  RR : BusSelector  Tag=PanoSim_System  OutputSignals=BodyKin_Wheel_Out_Bus.bodykin_whl_out_rr.xgnd_whl,BodyKin_Wheel_Out_Bus.bodykin_whl_out_rr.ygnd_whl,BodyKin_Wheel_Out_Bus.bodykin_whl_out_rr.zgnd_whl,BodyKin_Wheel_Out_Bus.bodykin_whl_out_rr.yaw_whl,BodyKin_Wheel_Out_Bus.bodykin_whl_out_rr.pitch_whl,BodyKin_Wheel_Out_Bus.bodykin_whl_out_rr.roll_whl,BodyKin_Wheel_Out_Bus.bodykin_whl_out_rr.vwx_whl,BodyKin_Wheel_Out_Bus.bodykin_whl_out_rr.vwy_whl,BodyKin_Wheel_Out_Bus.bodykin_whl_out_rr.vwz_whl,BodyKin_Wheel_Out_Bus.bodykin_whl_out_rr.rot_whl
  Scope1 : Scope
  Scope6 : Scope
  VehBusSelector3 : BusSelector  Tag=PanoSim_System  OutputSignals=Body_Out_Bus.Chassis_Motion.XO,Body_Out_Bus.Chassis_Motion.YO,Body_Out_Bus.Chassis_Motion.ZO,Body_Out_Bus.Chassis_Motion.YAW,Body_Out_Bus.Chassis_Motion.PITCH,Body_Out_Bus.Chassis_Motion.ROLL,Body_Out_Bus.Chassis_Motion.VX,Body_Out_Bus.Chassis_Motion.VY,Body_Out_Bus.Chassis_Motion.VZ,Body_Out_Bus.Chassis_Motion.AVZ,Body_Out_Bus.Chassis_Motion.AVY,Body_Out_Bus.Chassis_Motion.AVX,Body_Out_Bus.Chassis_Motion.AX,Body_Out_Bus.Chassis_Motion.AY,Body_Out_Bus.Chassis_Motion.AZ,Body_Out_Bus.Chassis_Motion.AAX,Body_Out_Bus.Chassis_Motion.AAY,Body_Out_Bus.Chassis_Motion.AAZ
  PlotBuilder_out : Outport
  wires:
  Bus Creator/1 -> PlotBuilder_out/1
  PowerandSteer/6 -> Demux/1  "<steer_str>"
  LF/9 -> Bus Creator/27  "<vwz_whl>"
  LF/6 -> Bus Creator/24  "<roll_whl>"
  F_LR/6 -> Bus Creator/84  "<mz_whl>"
  F_LR/5 -> Bus Creator/83  "<my_whl>"
  F_LR/3 -> Bus Creator/81  "<fz_whl>"
  Constant4/1 -> Bus Creator/53  "Rot_y_whl_l2"
  RF/9 -> Bus Creator/39  "<vwz_whl>"
  F_LR/2 -> Bus Creator/80  "<fy_whl>"
  RF/4 -> Bus Creator/34  "<yaw_whl>"
  RF/5 -> Bus Creator/35  "<pitch_whl>"
  LR/10 -> Bus Creator/52  "<rot_whl>"
  LR/9 -> Bus Creator/51  "<vwz_whl>"
  LR/8 -> Bus Creator/50  "<vwy_whl>"
  LR/6 -> Bus Creator/48  "<roll_whl>"
  LR/7 -> Bus Creator/49  "<vwx_whl>"
  LR/4 -> Bus Creator/46  "<yaw_whl>"
  LR/5 -> Bus Creator/47  "<pitch_whl>"
  LR/1 -> Bus Creator/43  "<xgnd_whl>"
  LR/2 -> Bus Creator/44  "<ygnd_whl>"
  PowerandSteer/5 -> Derivative/1  "<strav_sw>"
  VehBusSelector3/18 -> Bus Creator/18  "<AAZ>"
  RF/3 -> Bus Creator/33  "<zgnd_whl>"
  VehBusSelector3/17 -> Bus Creator/17  "<AAY>"
  Demux/4 -> Gain1/1
  VehBusSelector3/16 -> Bus Creator/16  "<AAX>"
  VehBusSelector3/14 -> Bus Creator/14  "<AY>"
  VehBusSelector3/13 -> Bus Creator/13  "<AX>"
  LF/4 -> Bus Creator/22  "<yaw_whl>"
  F_LF/6 -> Bus Creator/72  "<mz_whl>"
  F_LF/5 -> Bus Creator/71  "<my_whl>"
  F_LF/4 -> Bus Creator/70  "<mx_whl>"
  F_LF/3 -> Bus Creator/69  "<fz_whl>"
  F_LF/2 -> Bus Creator/68  "<fy_whl>"
  F_LF/1 -> Bus Creator/67  "<fx_whl>"
  RF/7 -> Bus Creator/37  "<vwx_whl>"
  RF/6 -> Bus Creator/36  "<roll_whl>"
  Constant1/1 -> Bus Creator/30  "Rot_z_whl_l1"
  F_RR/5 -> Bus Creator/89  "<my_whl>"
  RF/10 -> Bus Creator/40  "<rot_whl>"
  F_LR/1 -> Bus Creator/79  "<fx_whl>"
  F_RR/2 -> Bus Creator/86  "<fy_whl>"
  F_RR/1 -> Bus Creator/85  "<fx_whl>"
  Constant/1 -> Bus Creator/29  "Rot_y_whl_l1"
  F_RR/4 -> Bus Creator/88  "<mx_whl>"
  VehBusSelector3/5 -> Bus Creator/5  "<PITCH>"
  LF/8 -> Bus Creator/26  "<vwy_whl>"
  RR/4 -> Bus Creator/58  "<yaw_whl>"
  F_RR/3 -> Bus Creator/87  "<fz_whl>"
  VehBusSelector3/8 -> Bus Creator/8  "<VY>"
  RR/3 -> Bus Creator/57  "<zgnd_whl>"
  VehBusSelector3/11 -> Bus Creator/11  "<AVY>"
  RR/2 -> Bus Creator/56  "<ygnd_whl>"
  PowerandSteer/4 -> Gain2/1, Scope6/1  "<strav_sw>"
  Demux/3 -> Bus Creator/98  "Steer_lr_rad"
  F_RF/2 -> Bus Creator/74  "<fy_whl>"
  RR/1 -> Bus Creator/55  "<xgnd_whl>"
  F_RR/6 -> Bus Creator/90  "<mz_whl>"
  RR/10 -> Bus Creator/64  "<rot_whl>"
  Gain1/1 -> Bus Creator/99  "Steer_rr_rad"
  RR/7 -> Bus Creator/61  "<vwx_whl>"
  Constant7/1 -> Bus Creator/66  "Rot_z_whl_r2"
  F_RF/4 -> Bus Creator/76  "<mx_whl>"
  VehBusSelector3/6 -> Bus Creator/6  "<ROLL>"
  Constant3/1 -> Bus Creator/42  "Rot_z_whl_r1"
  Constant2/1 -> Bus Creator/41  "Rot_y_whl_r1"
  RR/9 -> Bus Creator/63  "<vwz_whl>"
  VehBusSelector3/1 -> Bus Creator/1  "<XO>"
  RR/8 -> Bus Creator/62  "<vwy_whl>"
  Constant6/1 -> Bus Creator/65  "Rot_y_whl_r2"
  VehBusSelector3/9 -> Bus Creator/9  "<VZ>"
  RR/6 -> Bus Creator/60  "<roll_whl>"
  Derivative/1 -> Scope1/1, Bus Creator/95  "Steerrate"
  VehBusSelector3/3 -> Bus Creator/3  "<ZO>"
  RF/1 -> Bus Creator/31  "<xgnd_whl>"
  RF/8 -> Bus Creator/38  "<vwy_whl>"
  Constant5/1 -> Bus Creator/54  "Rot_z_whl_l2"
  VehBusSelector3/10 -> Bus Creator/10  "<AVZ>"
  LF/1 -> Bus Creator/19  "<xgnd_whl>"
  F_RF/5 -> Bus Creator/77  "<my_whl>"
  PowerandSteer/2 -> Bus Creator/92  "<brake>"
  Gain2/1 -> Bus Creator/94  "Steerangle"
  VehicleDynOut/1 -> VehBusSelector3/1, LF/1, RF/1, LR/1, RR/1, F_LF/1, F_RF/1, F_LR/1, F_RR/1, PowerandSteer/1
  F_RF/6 -> Bus Creator/78  "<mz_whl>"
  VehBusSelector3/2 -> Bus Creator/2  "<YO>"
  Demux/2 -> Bus Creator/97  "Steer_rf_rad"
  LF/2 -> Bus Creator/20  "<ygnd_whl>"
  LF/7 -> Bus Creator/25  "<vwx_whl>"
  PowerandSteer/3 -> Bus Creator/93  "<pt_gear_status>"
  VehBusSelector3/7 -> Bus Creator/7  "<VX>"
  LR/3 -> Bus Creator/45  "<zgnd_whl>"
  VehBusSelector3/15 -> Bus Creator/15  "<AZ>"
  VehBusSelector3/4 -> Bus Creator/4  "<YAW>"
  Gain/1 -> Bus Creator/96  "Steer_lf_rad"
  RR/5 -> Bus Creator/59  "<pitch_whl>"
  PowerandSteer/1 -> Bus Creator/91  "<pt_throttle>"
  LF/5 -> Bus Creator/23  "<pitch_whl>"
  F_LR/4 -> Bus Creator/82  "<mx_whl>"
  F_RF/3 -> Bus Creator/75  "<fz_whl>"
  LF/10 -> Bus Creator/28  "<rot_whl>"
  RF/2 -> Bus Creator/32  "<ygnd_whl>"
  Demux/1 -> Gain/1
  VehBusSelector3/12 -> Bus Creator/12  "<AVX>"
  LF/3 -> Bus Creator/21  "<zgnd_whl>"
  F_RF/1 -> Bus Creator/73  "<fx_whl>"

== system AVW_b/Veh_1/Veh_1_Sensors ==
  note: Help
  In1 : Inport
  OBU_BSM : Subsystem  Tag=PanoSim_System
      mask Display: image(imread('V2X.png'));
  SensorBus : BusCreator  Inputs=1
  Out1 : Outport
  wires:
  SensorBus/1 -> Out1/1
  In1/1 -> OBU_BSM/1(In1)
  OBU_BSM/1(Out1) -> SensorBus/1  "OBU_BSM_Out"

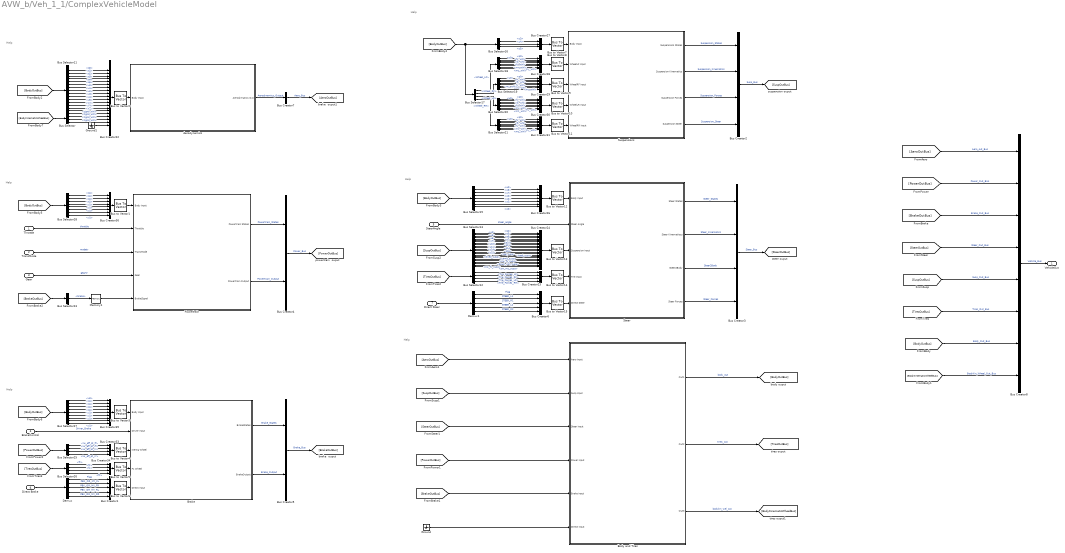
== system AVW_b/Veh_1_1/ComplexVehicleModel ==
  note: Help
  note: Help
  note: Help
  note: Help
  note: Help
  note: Help
  Throttle : Inport
  TransMode : Inport  Port=2
  Gear : Inport  Port=3
  BrakeControl : Inport  Port=4
  SteerAngle : Inport  Port=5
  Direct Brake : Inport  Port=6
  Direct Steer : Inport  Port=7
  Aerodynamics : Subsystem
  Body and Tires : Subsystem
  Brake : Subsystem
  Bus Creator1 : BusCreator  Inputs=5
  Bus Creator{2..3,23,33..34} (5 alike) : BusCreator  Inputs=4
  Bus Creator22 : BusCreator  Inputs=20
  Bus Creator24 : BusCreator  Inputs=24
  Bus Creator26 : BusCreator  Inputs=7
  Bus Creator27 : BusCreator  Inputs=3
  Bus Creator{8,28..31,36} (6 alike) : BusCreator  Inputs=8
  Bus Creator35 : BusCreator  Inputs=9
  Bus Creator4 : BusCreator  Inputs=2
  Bus Creator5 : BusCreator  Inputs=2
  Bus Creator6 : BusCreator  Inputs=5
  Bus Creator7 : BusCreator  Inputs=1
  Bus Selector : BusSelector  OutputSignals=bodykin_whl_out_lf.zgnd_whl,bodykin_whl_out_rf.zgnd_whl,bodykin_whl_out_lr.zgnd_whl,bodykin_whl_out_rr.zgnd_whl
  Bus Selector11 : BusSelector  OutputSignals=Chassi_States.q0,Chassi_States.q1,Chassi_States.q2,Chassi_States.q3,Chassi_States.q4,Chassi_States.q5,Chassi_States.u0,Chassi_States.u1,Chassi_States.u2,Chassi_States.u3,Chassi_States.u4,Chassi_States.u5,Chassis_Motion.VX,Chassis_Motion.VY,Chassis_Motion.VZ
  Bus Selector12 : BusSelector  OutputSignals=Tire_Forces_LF,Tire_Forces_RF,Tire_Forces_LR,Tire_Forces_RR
  Bus Selector13 : BusSelector  OutputSignals=Suspension_States.q2,Suspension_States.u2,Suspension_States.q3,Suspension_States.u3,Suspension_States.q6,Suspension_States.u6,Suspension_States.q7,Suspension_States.u7,Suspension_States.q10,Suspension_States.u10,Suspension_States.q11,Suspension_States.u11,Suspension_States.q14,Suspension_States.u14,Suspension_States.q15,Suspension_States.u15,Suspension_Kinematics.toe_susp,Suspension_Kinematics.toed_susp,Suspension_Kinematics.dived_susp,Suspension_Kinematics.camd_susp,Suspension_Kinematics.dcam_con_susp,Suspension_Steer.sw_fx_susp,Suspension_Steer.sw_fy_susp,Suspension_Steer.sw_mz_susp
  Bus Selector15 : BusSelector  OutputSignals=Chassi_States.u0,Chassi_States.u6,Chassi_States.u7,Wheel_LF.u0,Wheel_RF.u0,Wheel_LR.u0,Wheel_RR.u0
  Bus Selector16 : BusSelector  OutputSignals=Chassi_States.u3,Chassi_States.u4,Chassi_States.u5
  Bus Selector17 : BusSelector  OutputSignals=Wheel_LF,Wheel_RF,Wheel_LR,Wheel_RR
  Bus Selector{18..21} (4 alike) : BusSelector  OutputSignals=q0,u0,fx_whl,fy_whl,fz_whl,mx_whl,my_whl,mz_whl
  Bus Selector23 : BusSelector  OutputSignals=Brake_Output.brake
  Bus Selector25 : BusSelector  OutputSignals=Powertrain_Output.iw_eff_pt_lf,Powertrain_Output.iw_eff_pt_rf,Powertrain_Output.iw_eff_pt_lr,Powertrain_Output.iw_eff_pt_rr
  Bus Selector26 : BusSelector  OutputSignals=Tire_Forces_LF.fz,Tire_Forces_RF.fz,Tire_Forces_LR.fz,Tire_Forces_RR.fz
  Bus Selector27 : BusSelector  OutputSignals=Chassi_States.u0,Wheel_LF.q1,Wheel_RF.q1,Wheel_LR.q1,Wheel_RR.q1,Wheel_LF.u1,Wheel_RF.u1,Wheel_LR.u1,Wheel_RR.u1
  Bus Selector28 : BusSelector  OutputSignals=Wheel_LF.q1,Wheel_RF.q1,Wheel_LR.q1,Wheel_RR.q1,Wheel_LF.u1,Wheel_RF.u1,Wheel_LR.u1,Wheel_RR.u1
  Bus to Vector{1..15} (15 alike) : BusToVector
  Demux : Demux  Outputs=5
  Demux1 : Demux  Outputs=5
  Ground : Ground
  Ground1 : Ground
  Memory1 : Memory
  Powertrain : Subsystem
  Steer : Subsystem
  Suspensions : Subsystem
  VehicleOut : Outport
  wires:
  Ground/1 -> Body and Tires/6(Direct Input)
  Bus Selector13/24 -> Bus Creator24/24  "<sw_mz_susp>"
  Bus Selector13/23 -> Bus Creator24/23  "<sw_fy_susp>"
  Bus Selector13/22 -> Bus Creator24/22  "<sw_fx_susp>"
  Bus Selector13/21 -> Bus Creator24/21  "<dcam_con_susp>"
  Bus Selector13/20 -> Bus Creator24/20  "<camd_susp>"
  Bus Selector13/19 -> Bus Creator24/19  "<dived_susp>"
  Bus Selector13/18 -> Bus Creator24/18  "<toed_susp>"
  Bus Selector13/17 -> Bus Creator24/17  "<toe_susp>"
  Bus Selector13/16 -> Bus Creator24/16  "<u15>"
  Bus Selector13/15 -> Bus Creator24/15  "<q15>"
  Bus Selector13/14 -> Bus Creator24/14  "<u14>"
  Bus Selector13/13 -> Bus Creator24/13  "<q14>"
  Bus Selector13/12 -> Bus Creator24/12  "<u11>"
  Bus Selector13/11 -> Bus Creator24/11  "<q11>"
  Bus Selector13/10 -> Bus Creator24/10  "<u10>"
  Bus Selector13/9 -> Bus Creator24/9  "<q10>"
  Bus Selector13/8 -> Bus Creator24/8  "<u7>"
  Bus Selector13/7 -> Bus Creator24/7  "<q7>"
  Bus Selector13/6 -> Bus Creator24/6  "<u6>"
  Bus Selector13/5 -> Bus Creator24/5  "<q6>"
  Bus Selector13/4 -> Bus Creator24/4  "<u3>"
  Bus Selector13/3 -> Bus Creator24/3  "<q3>"
  Bus Selector13/2 -> Bus Creator24/2  "<u2>"
  Bus Selector13/1 -> Bus Creator24/1  "<q2>"
  Demux1/5 -> Bus Creator6/5  "STEER_R2"
  Demux1/4 -> Bus Creator6/4  "STEER_L2"
  Demux1/3 -> Bus Creator6/3  "STEER_R1"
  Demux1/2 -> Bus Creator6/2  "STEER_L1"
  Demux1/1 -> Bus Creator6/1  "Flag"
  Direct Steer/1 -> Demux1/1
  Bus Creator6/1 -> Bus to Vector15/1
  Demux/5 -> Bus Creator1/5  "PBK_OR_MY_RR"
  Demux/4 -> Bus Creator1/4  "PBK_OR_MY_RL"
  Demux/3 -> Bus Creator1/3  "PBK_OR_MY_FR"
  Demux/2 -> Bus Creator1/2  "PBK_OR_MY_FL"
  Demux/1 -> Bus Creator1/1  "Flag"
  Direct Brake/1 -> Demux/1
  SteerAngle/1 -> Steer/2(Steer Angle)  "steer_angle"
  [TiresOutBus] -> Bus Creator8/6  "Tires_Out_Bus"
  [SuspOutBus] -> Bus Creator8/5  "Susp_Out_Bus"
  [SteerOutBus] -> Bus Creator8/4  "Steer_Out_Bus"
  [BrakeOutBus] -> Bus Creator8/3  "Brake_Out_Bus"
  [PowerOutBus] -> Bus Creator8/2  "Power_Out_BUs"
  [AeroOutBus] -> Bus Creator8/1  "Aero_out_Bus"
  Suspensions/4(Suspension Steer) -> Bus Creator2/4  "Suspension_Steer"
  Suspensions/3(Suspension Forces) -> Bus Creator2/3  "Suspension_Forces"
  Suspensions/1(Suspensions States) -> Bus Creator2/1  "Suspension_States"
  Suspensions/2(Suspension Kinematics) -> Bus Creator2/2  "Suspension_Kinematics"
  Bus Creator2/1 -> [SuspOutBus]  "Susp_Bus"
  Steer/1(Steer States) -> Bus Creator3/1  "Steer_States"
  Steer/2(Steer Kinematiocs) -> Bus Creator3/2  "Steer_Kinematics"
  Steer/3(Steer2Body) -> Bus Creator3/3  "Steer2Body"
  Steer/4(Steer Forces) -> Bus Creator3/4  "Steer_Forces"
  Bus Creator3/1 -> [SteerOutBus]  "Steer_Bus"
  Powertrain/1(Powertrain States) -> Bus Creator4/1  "Powertrain_States"
  Powertrain/2(Powertrain Output) -> Bus Creator4/2  "Powertrain_Output"
  Bus Creator4/1 -> [PowerOutBus]  "Power_Bus"
  Brake/1(BrakeStates) -> Bus Creator5/1  "Brake_States"
  Brake/2(BrakeOutput) -> Bus Creator5/2  "Brake_Output"
  Bus Creator5/1 -> [BrakeOutBus]  "Brake_Bus"
  Aerodynamics/1(Aerodymatics Out) -> Bus Creator7/1  "Aerodynamics_Output"
  Bus Creator7/1 -> [AeroOutBus]  "Aero_Bus"
  Bus Creator8/1 -> VehicleOut/1  "Vehicle_Bus"
  [BodyOutBus] -> Bus Creator8/7  "Body_Out_Bus"
  [BodyOutBus] -> Bus Selector11/1
  [TiresOutBus] -> Bus Selector12/1
  Bus Selector12/1 -> Bus Creator23/1  "<Tire_Forces_LF>"
  Bus Selector12/2 -> Bus Creator23/2  "<Tire_Forces_RF>"
  Bus Selector12/3 -> Bus Creator23/3  "<Tire_Forces_LR>"
  Bus Selector12/4 -> Bus Creator23/4  "<Tire_Forces_RR>"
  [SuspOutBus] -> Bus Selector13/1
  Bus Creator24/1 -> Bus to Vector13/1
  [BodyOutBus] -> Bus Selector15/1
  Bus Selector15/1 -> Bus Creator26/1  "<u0>"
  Bus Selector15/2 -> Bus Creator26/2  "<u6>"
  Bus Selector15/3 -> Bus Creator26/3  "<u7>"
  Bus Selector15/4 -> Bus Creator26/4  "<u0>"
  Bus Selector15/5 -> Bus Creator26/5  "<u0>"
  Bus Selector15/6 -> Bus Creator26/6  "<u0>"
  Bus Selector15/7 -> Bus Creator26/7  "<u0>"
  Bus Selector16/1 -> Bus Creator27/1  "<u3>"
  Bus Selector16/2 -> Bus Creator27/2  "<u4>"
  Bus Selector16/3 -> Bus Creator27/3  "<u5>"
  Bus Creator27/1 -> Bus to Vector7/1
  Bus Selector17/1 -> Bus Selector18/1  "<Wheel_LF>"
  Bus Selector18/1 -> Bus Creator28/1  "<q0>"
  Bus Selector18/2 -> Bus Creator28/2  "<u0>"
  Bus Selector18/3 -> Bus Creator28/3  "<fx_whl>"
  Bus Selector18/4 -> Bus Creator28/4  "<fy_whl>"
  Bus Selector18/5 -> Bus Creator28/5  "<fz_whl>"
  Bus Selector18/6 -> Bus Creator28/6  "<mx_whl>"
  Bus Selector18/7 -> Bus Creator28/7  "<my_whl>"
  Bus Selector18/8 -> Bus Creator28/8  "<mz_whl>"
  Bus Selector19/1 -> Bus Creator29/1  "<q0>"
  Bus Selector19/2 -> Bus Creator29/2  "<u0>"
  Bus Selector19/3 -> Bus Creator29/3  "<fx_whl>"
  Bus Selector19/4 -> Bus Creator29/4  "<fy_whl>"
  Bus Selector19/5 -> Bus Creator29/5  "<fz_whl>"
  Bus Selector19/6 -> Bus Creator29/6  "<mx_whl>"
  Bus Selector19/7 -> Bus Creator29/7  "<my_whl>"
  Bus Selector19/8 -> Bus Creator29/8  "<mz_whl>"
  Bus Selector20/1 -> Bus Creator30/1  "<q0>"
  Bus Selector20/2 -> Bus Creator30/2  "<u0>"
  Bus Selector20/3 -> Bus Creator30/3  "<fx_whl>"
  Bus Selector20/4 -> Bus Creator30/4  "<fy_whl>"
  Bus Selector20/5 -> Bus Creator30/5  "<fz_whl>"
  Bus Selector20/6 -> Bus Creator30/6  "<mx_whl>"
  Bus Selector20/7 -> Bus Creator30/7  "<my_whl>"
  Bus Selector20/8 -> Bus Creator30/8  "<mz_whl>"
  Bus Selector21/1 -> Bus Creator31/1  "<q0>"
  Bus Selector21/2 -> Bus Creator31/2  "<u0>"
  Bus Selector21/3 -> Bus Creator31/3  "<fx_whl>"
  Bus Selector21/4 -> Bus Creator31/4  "<fy_whl>"
  Bus Selector21/5 -> Bus Creator31/5  "<fz_whl>"
  Bus Selector21/6 -> Bus Creator31/6  "<mx_whl>"
  Bus Selector21/7 -> Bus Creator31/7  "<my_whl>"
  Bus Selector21/8 -> Bus Creator31/8  "<mz_whl>"
  Bus Selector17/2 -> Bus Selector19/1  "<Wheel_RF>"
  Bus Selector17/3 -> Bus Selector20/1  "<Wheel_LR>"
  Bus Selector17/4 -> Bus Selector21/1  "<Wheel_RR>"
  Bus Creator28/1 -> Bus to Vector8/1
  Bus Creator29/1 -> Bus to Vector9/1
  Bus Creator30/1 -> Bus to Vector10/1
  Bus Creator31/1 -> Bus to Vector11/1
  Throttle/1 -> Powertrain/2(Throttle)  "throttle"
  TransMode/1 -> Powertrain/3(TransMode)  "modetr"
  Gear/1 -> Powertrain/4(Gear)  "geartr"
  [BrakeOutBus] -> Bus Selector23/1
  BrakeControl/1 -> Brake/2(Driver Input)  "Driver_Brake"
  [PowerOutBus] -> Bus Selector25/1
  Bus Selector25/1 -> Bus Creator33/1  "<iw_eff_pt_lf>"
  Bus Selector25/2 -> Bus Creator33/2  "<iw_eff_pt_rf>"
  Bus Selector25/3 -> Bus Creator33/3  "<iw_eff_pt_lr>"
  Bus Selector25/4 -> Bus Creator33/4  "<iw_eff_pt_rr>"
  [TiresOutBus] -> Bus Selector26/1
  Bus Selector26/1 -> Bus Creator34/1  "<fz>"
  Bus Selector26/2 -> Bus Creator34/2  "<fz>"
  Bus Selector26/3 -> Bus Creator34/3  "<fz>"
  Bus Selector26/4 -> Bus Creator34/4  "<fz>"
  [BodyOutBus] -> Bus Selector27/1
  Bus Selector27/1 -> Bus Creator35/1  "<u0>"
  Bus Selector27/2 -> Bus Creator35/2  "<q1>"
  Bus Selector27/3 -> Bus Creator35/3  "<q1>"
  Bus Selector27/4 -> Bus Creator35/4  "<q1>"
  Bus Selector27/5 -> Bus Creator35/5  "<q1>"
  Bus Selector27/6 -> Bus Creator35/6  "<u1>"
  Bus Selector27/7 -> Bus Creator35/7  "<u1>"
  Bus Selector27/8 -> Bus Creator35/8  "<u1>"
  Bus Selector27/9 -> Bus Creator35/9  "<u1>"
  [BodyOutBus] -> Bus Selector28/1
  Bus Selector28/1 -> Bus Creator36/1  "<q1>"
  Bus Selector28/2 -> Bus Creator36/2  "<q1>"
  Bus Selector28/3 -> Bus Creator36/3  "<q1>"
  Bus Selector28/4 -> Bus Creator36/4  "<q1>"
  Bus Selector28/5 -> Bus Creator36/5  "<u1>"
  Bus Selector28/6 -> Bus Creator36/6  "<u1>"
  Bus Selector28/7 -> Bus Creator36/7  "<u1>"
  Bus Selector28/8 -> Bus Creator36/8  "<u1>"
  Bus Selector11/1 -> Bus Creator22/1  "<q0>"
  Bus Selector11/2 -> Bus Creator22/2  "<q1>"
  Bus Selector11/3 -> Bus Creator22/3  "<q2>"
  Bus Selector11/4 -> Bus Creator22/4  "<q3>"
  Bus Selector11/5 -> Bus Creator22/5  "<q4>"
  Bus Selector11/6 -> Bus Creator22/6  "<q5>"
  Bus Selector11/7 -> Bus Creator22/7  "<u0>"
  Bus Selector11/8 -> Bus Creator22/8  "<u1>"
  Bus Selector11/9 -> Bus Creator22/9  "<u2>"
  Bus Selector11/10 -> Bus Creator22/10  "<u3>"
  Bus Selector11/11 -> Bus Creator22/11  "<u4>"
  Bus Selector11/12 -> Bus Creator22/12  "<u5>"
  Bus Selector11/13 -> Bus Creator22/13  "<VX>"
  Bus Selector11/14 -> Bus Creator22/14  "<VY>"
  Bus Selector11/15 -> Bus Creator22/15  "<VZ>"
  Ground1/1 -> Bus Creator22/20
  [SteerOutBus] -> Body and Tires/3(Steer Input)
  [PowerOutBus] -> Body and Tires/4(Power Input)
  Body and Tires/1(Out1) -> [BodyOutBus]  "body_out"
  Body and Tires/2(Out2) -> [TiresOutBus]  "tires_out"
  [AeroOutBus] -> Body and Tires/1(Aero Input)
  [SuspOutBus] -> Body and Tires/2(Susp Input)
  Bus Selector23/1 -> Memory1/1  "<brake>"
  Memory1/1 -> Powertrain/5(BrakeSignal)
  Bus Creator26/1 -> Bus to Vector12/1
  Bus Creator23/1 -> Bus to Vector14/1
  Bus Creator36/1 -> Bus to Vector1/1
  [BodyOutBus] -> Bus Selector16/1, Bus Selector17/1
  [BrakeOutBus] -> Body and Tires/5(Brake Input)
  Body and Tires/3(Out3) -> [BodyKinematicWheelBus]  "bodykin_wel_out"
  [BodyKinematicWheelBus] -> Bus Creator8/8  "BodyKin_Wheel_Out_Bus"
  [BodyKinematicWheelBus] -> Bus Selector/1
  Bus Selector/1 -> Bus Creator22/16  "<zgnd_whl>"
  Bus Selector/2 -> Bus Creator22/17  "<zgnd_whl>"
  Bus Selector/3 -> Bus Creator22/18  "<zgnd_whl>"
  Bus Selector/4 -> Bus Creator22/19  "<zgnd_whl>"
  Bus Creator22/1 -> Bus to Vector2/1
  Bus to Vector2/1 -> Aerodynamics/1(Body Input)
  Bus to Vector1/1 -> Powertrain/1(Body Input)
  Bus Creator35/1 -> Bus to Vector3/1
  Bus to Vector3/1 -> Brake/1(Body Input)
  Bus Creator33/1 -> Bus to Vector4/1
  Bus to Vector4/1 -> Brake/3(Inertia Wheel)
  Bus Creator34/1 -> Bus to Vector5/1
  Bus to Vector5/1 -> Brake/4(Fz Wheel)
  Bus Creator1/1 -> Bus to Vector6/1
  Bus to Vector6/1 -> Brake/5(Direct Input)
  Bus to Vector7/1 -> Suspensions/1(Body Input)
  Bus to Vector8/1 -> Suspensions/2(WheelLF Input)
  Bus to Vector9/1 -> Suspensions/3(WheelRF Input)
  Bus to Vector10/1 -> Suspensions/4(WheelLR Input)
  Bus to Vector11/1 -> Suspensions/5(WheelRR Input)
  Bus to Vector12/1 -> Steer/1(Body Input)
  Bus to Vector13/1 -> Steer/3(Suspension Input)
  Bus to Vector14/1 -> Steer/4(Tire Input)
  Bus to Vector15/1 -> Steer/5(Direct Steer)
